simulink subsystem "Translation"  (R2023a)
settings: Solver=VariableStepAuto  StartTime=0.0  StopTime=10.0  RelTol=1e-3
values from neighbouring files (symbols this model uses):
  G = [0 ; 0 ; m*g]    [constants.m]
  k = 3.1582e-10    [constants.m]
  m = 28.6e-3    (= 0.0286)    [constants.m]
settings Model: Creator=raphb  LastModifiedBy=raphb

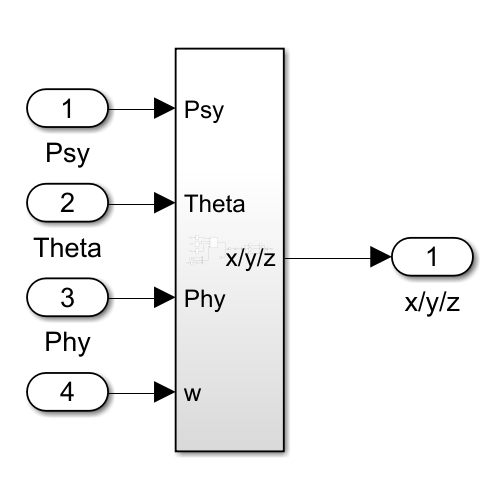
[thumbnail: Simulink's stored preview of the top-level diagram]
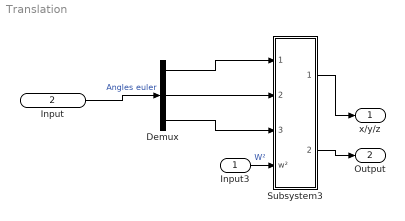
== system Translation ==
  Input3 : Inport
  Input : Inport  Port=2
  Demux : Demux  Outputs=3
  Subsystem3 : Subsystem
  x/y/z : Outport
  Output : Outport  Port=2
  wires:
  Subsystem3/1(x/y/z) -> x/y/z/1
  Input3/1 -> Subsystem3/4(w²)  "W²"
  Input/1 -> Demux/1  "Angles euler"
  Demux/1 -> Subsystem3/1(Phi)
  Demux/2 -> Subsystem3/2(Theta)
  Demux/3 -> Subsystem3/3(Psy)
  Subsystem3/2(derivees) -> Output/1

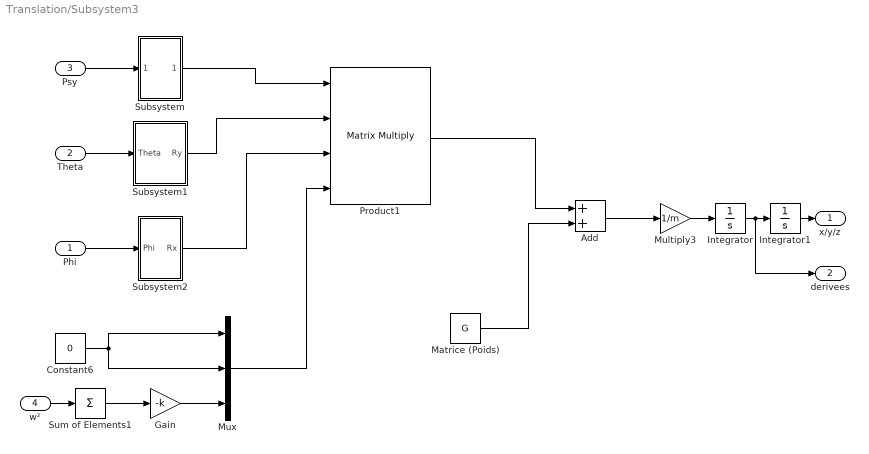
== system Translation/Subsystem3 ==
  Phi : Inport
  Theta : Inport  Port=2
  Psy : Inport  Port=3
  w² : Inport  Port=4
  Add : Sum
  Constant6 : Constant  Value=0
  Gain : Gain  Gain=-k
  Integrator : Integrator
  Integrator1 : Integrator  InitialCondition=[0, 0, -1]
  Matrice (Poids) : Constant  Value=G
  Multiply3 : Gain  Gain=1/m
  Mux : Mux  Inputs=3
  Product1 : Product  Inputs=4  Multiplication=Matrix(*)
  Subsystem : Subsystem
  Subsystem1 : Subsystem
  Subsystem2 : Subsystem
  Sum of Elements1 : Sum  Inputs=+
  x/y/z : Outport
  derivees : Outport  Port=2
  wires:
  Integrator1/1 -> x/y/z/1
  Integrator/1 -> Integrator1/1, derivees/1
  Multiply3/1 -> Integrator/1
  Matrice (Poids)/1 -> Add/2
  Subsystem/1(Out1) -> Product1/1
  Subsystem1/1(Ry) -> Product1/2
  Constant6/1 -> Mux/1, Mux/2
  Product1/1 -> Add/1
  Phi/1 -> Subsystem2/1(Phi)
  Psy/1 -> Subsystem/1(Psy)
  Add/1 -> Multiply3/1
  Mux/1 -> Product1/4
  Theta/1 -> Subsystem1/1(Theta)
  Subsystem2/1(Rx) -> Product1/3
  Gain/1 -> Mux/3
  Sum of Elements1/1 -> Gain/1
  w²/1 -> Sum of Elements1/1

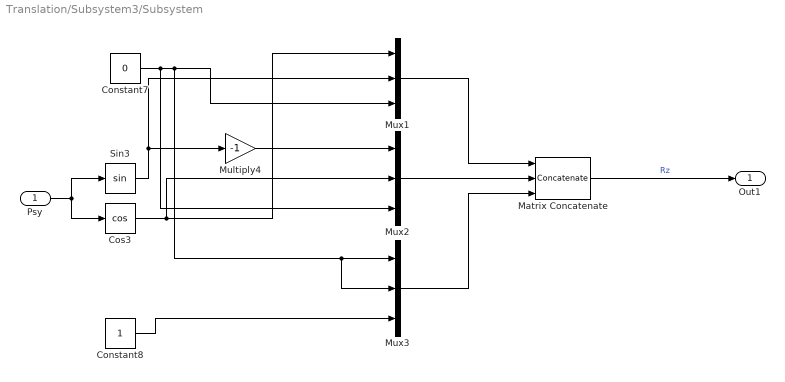
== system Translation/Subsystem3/Subsystem ==
  Psy : Inport
  Constant7 : Constant  Value=0
  Constant8 : Constant
  Cos3 : Trigonometry  Operator=cos
  Matrix Concatenate : Concatenate  NumInputs=3  Mode=Multidimensional array  ConcatenateDimension=2
  Multiply4 : Gain  Gain=-1
  Mux1 : Mux  Inputs=3
  Mux2 : Mux  Inputs=3
  Mux3 : Mux  Inputs=3
  Sin3 : Trigonometry
  Out1 : Outport
  wires:
  Sin3/1 -> Multiply4/1, Mux1/2
  Psy/1 -> Sin3/1, Cos3/1
  Mux2/1 -> Matrix Concatenate/2
  Mux1/1 -> Matrix Concatenate/1
  Mux3/1 -> Matrix Concatenate/3
  Matrix Concatenate/1 -> Out1/1  "Rz"
  Cos3/1 -> Mux2/2, Mux1/1
  Constant7/1 -> Mux2/3, Mux3/1, Mux3/2, Mux1/3
  Multiply4/1 -> Mux2/1
  Constant8/1 -> Mux3/3

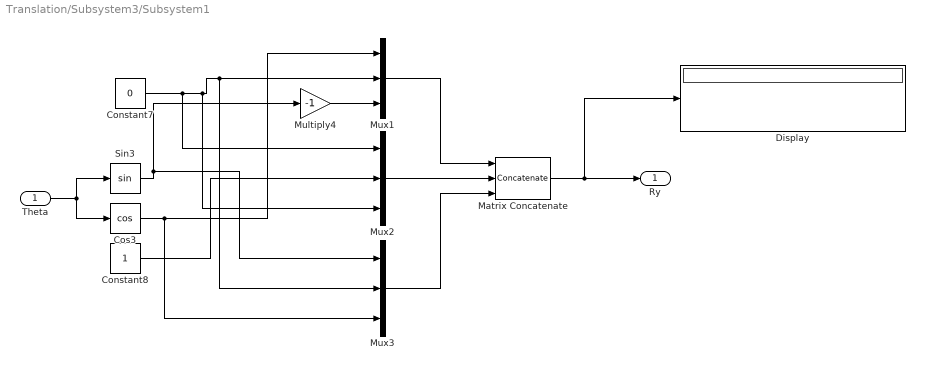
== system Translation/Subsystem3/Subsystem1 ==
  Theta : Inport
  Constant7 : Constant  Value=0
  Constant8 : Constant
  Cos3 : Trigonometry  Operator=cos
  Display : Display
  Matrix Concatenate : Concatenate  NumInputs=3  Mode=Multidimensional array  ConcatenateDimension=2
  Multiply4 : Gain  Gain=-1
  Mux1 : Mux  Inputs=3
  Mux2 : Mux  Inputs=3
  Mux3 : Mux  Inputs=3
  Sin3 : Trigonometry
  Ry : Outport
  wires:
  Theta/1 -> Sin3/1, Cos3/1
  Sin3/1 -> Mux3/1, Multiply4/1
  Mux2/1 -> Matrix Concatenate/2
  Mux3/1 -> Matrix Concatenate/3
  Mux1/1 -> Matrix Concatenate/1
  Cos3/1 -> Mux3/3, Mux1/1
  Constant7/1 -> Mux2/1, Mux2/3, Mux3/2, Mux1/2
  Multiply4/1 -> Mux1/3
  Constant8/1 -> Mux2/2
  Matrix Concatenate/1 -> Display/1, Ry/1

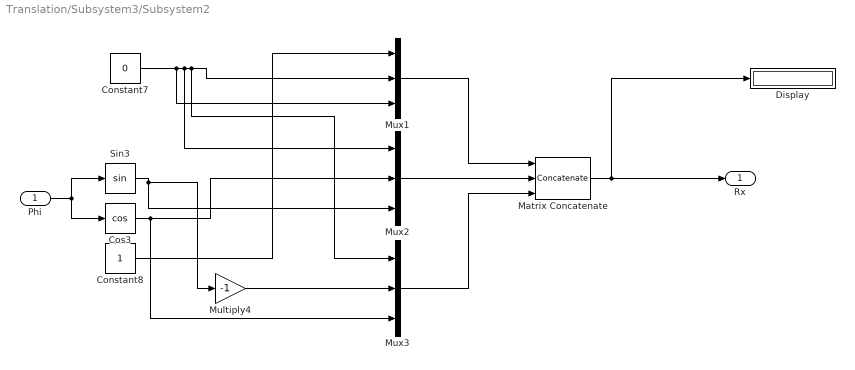
== system Translation/Subsystem3/Subsystem2 ==
  Phi : Inport
  Constant7 : Constant  Value=0
  Constant8 : Constant
  Cos3 : Trigonometry  Operator=cos
  Display : Display
  Matrix Concatenate : Concatenate  NumInputs=3  Mode=Multidimensional array  ConcatenateDimension=2
  Multiply4 : Gain  Gain=-1
  Mux1 : Mux  Inputs=3
  Mux2 : Mux  Inputs=3
  Mux3 : Mux  Inputs=3
  Sin3 : Trigonometry
  Rx : Outport
  wires:
  Sin3/1 -> Multiply4/1, Mux2/3
  Phi/1 -> Sin3/1, Cos3/1
  Mux2/1 -> Matrix Concatenate/2
  Mux1/1 -> Matrix Concatenate/1
  Mux3/1 -> Matrix Concatenate/3
  Matrix Concatenate/1 -> Display/1, Rx/1
  Constant8/1 -> Mux1/1
  Constant7/1 -> Mux1/3, Mux2/1, Mux3/1, Mux1/2
  Cos3/1 -> Mux3/3, Mux2/2
  Multiply4/1 -> Mux3/2
